simulink subsystem "FFT"  (R2020b)
settings: Solver=VariableStepAuto  StartTime=0.0  StopTime=10.0  RelTol=1e-3
values from neighbouring files (symbols this model uses):
  params = bestParams    [trainNet.m]
libraries: simulink x2, dsphdlxfrm x1
settings Model: Creator=trevor  LastModifiedBy=trevor
settings DebuggingCC: SFMachineParentedDataDiag=error

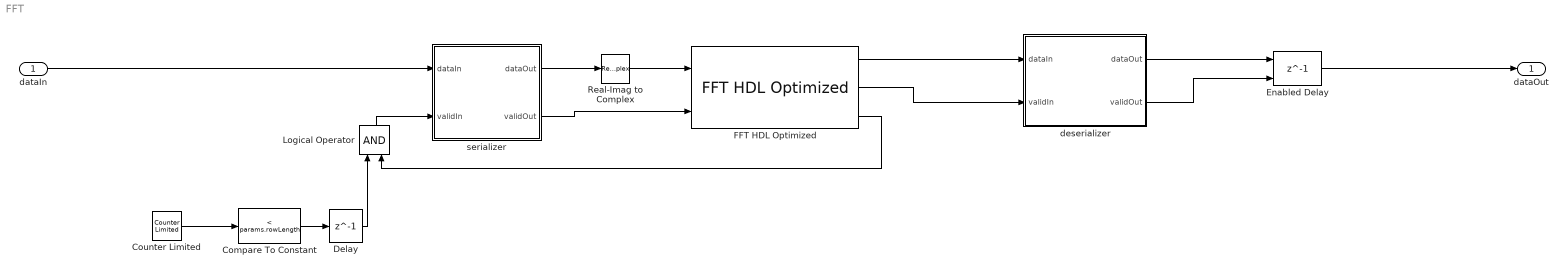
== system FFT ==
  dataIn : Inport
  Compare To Constant : simulink/Logic and Bit Operations/Compare To Constant  relop=<  const=params.rowLength  OutDataTypeStr=boolean
  Counter Limited : simulink/Sources/Counter Limited  uplimit=params.samplingPeriod/params.systemClockPeriod  tsamp=-1
  Delay : Delay  DelayLength=1
  Enabled Delay : Delay  DelayLength=1  ShowEnablePort=on
      settings: InputPortMap=u0,e6
  FFT HDL Optimized : dsphdlxfrm/FFT HDL Optimized  FFTLength=params.FFTSize  Architecture=Burst Radix 2  ComplexMultiplication=Use 4 multipliers and 2 adders  BitReversedOutput=off  BitReversedInput=off  Normalize=off  SimulateUsing=Code generation  RoundingMethod=Floor  ResetInputPort=off  StartOutputPort=off  EndOutputPort=off
      settings: SourceProductBaseCode=DS
  Logical Operator : Logic  AllPortsSameDT=off  OutDataTypeStr=boolean
  Real-Imag to Complex : RealImagToComplex  Input=Real
  deserializer : MATLAB Function  TreatAsAtomicUnit=on
  serializer : MATLAB Function  TreatAsAtomicUnit=on
  dataOut : Outport
  wires:
  serializer/1(dataOut) -> Real-Imag to Complex/1
  serializer/2(validOut) -> FFT HDL Optimized/2
  FFT HDL Optimized/2 -> deserializer/2(validIn)
  FFT HDL Optimized/1 -> deserializer/1(dataIn)
  deserializer/2(validOut) -> Enabled Delay/2
  deserializer/1(dataOut) -> Enabled Delay/1
  Real-Imag to Complex/1 -> FFT HDL Optimized/1
  Enabled Delay/1 -> dataOut/1
  dataIn/1 -> serializer/1(dataIn)
  Counter Limited/1 -> Compare To Constant/1
  Compare To Constant/1 -> Delay/1
  FFT HDL Optimized/3 -> Logical Operator/2
  Logical Operator/1 -> serializer/2(validIn)
  Delay/1 -> Logical Operator/1

== matlab function FFT/deserializer ==
  settings: fimath=fimath('RoundingMethod', 'Floor','OverflowAction', 'Wrap','ProductMode', 'FullPrecision', 'SumMode', 'FullPrecision')
  data: dataOut output; dataIn input; validOut output; validIn input
function [dataOut, validOut] = deserialize(dataIn, validIn)
%#codegen

persistent shiftReg
if isempty(shiftReg)
    shiftReg = zeros(1,1024, 'like', dataIn);
end

persistent wordCount
if isempty(wordCount)
    wordCount = ufi(0, 10, 0);
end

if validIn
    shiftReg(1:1023) = shiftReg(2:1024);
    shiftReg(1024) = dataIn;
    
    
    if wordCount == cast(1023, 'like', wordCount)
        wordCount = cast(0, 'like', wordCount);
        validOut = true;
    else
        wordCount(:) = wordCount + cast(1, 'like', wordCount);
        validOut = false;
    end
else
    validOut = false;
end

dataOut = shiftReg;

== matlab function FFT/serializer ==
  settings: fimath=fimath('RoundingMethod', 'Floor','OverflowAction', 'Wrap','ProductMode', 'FullPrecision', 'SumMode', 'FullPrecision')
  data: dataIn input; dataOut output; validIn input boolean; validOut output boolean
function [dataOut, validOut] = serialize(dataIn, validIn)
%#codegen

persistent wordCount
if isempty(wordCount)
    wordCount = ufi(0, 10, 0);
end

if validIn
        dataOut = dataIn(wordCount + 1);
        validOut = true;
        
        if wordCount == cast(1023, 'like', wordCount)
            wordCount = cast(0, 'like', wordCount);
        else
            wordCount(:) = wordCount + cast(1, 'like', wordCount);
        end
else
    validOut = false;
    dataOut = cast(0, 'like', dataIn);
end
